simulink subsystem "CA"  (R2025a)
settings: Solver=VariableStepAuto  StartTime=0.0  StopTime=10.0  RelTol=1e-3
libraries: px4Utilslib x12
settings Model: Creator=gurt1  LastModifiedBy=gurt1

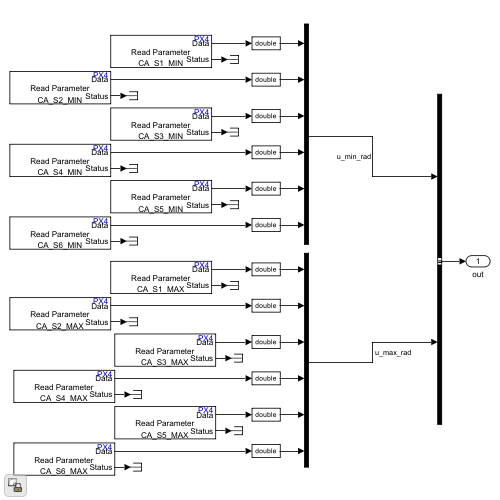
[thumbnail: Simulink's stored preview of the top-level diagram]
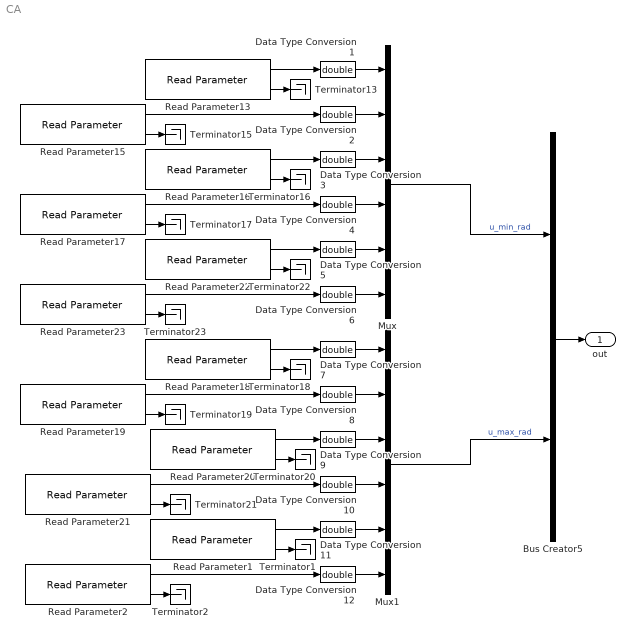
== system CA ==
  Bus Creator5 : BusCreator  Inputs=2
  Data Type Conversion{1..12} (12 alike) : DataTypeConversion  OutDataTypeStr=double  SaturateOnIntegerOverflow=off  RndMeth=Floor
  Mux : Mux  Inputs=6
  Mux1 : Mux  Inputs=6
  Read Parameter1 : px4Utilslib/Read Parameter  ParameterName=CA_S5_MAX  DataType=FLOAT  SampleTime=-1
  Read Parameter13 : px4Utilslib/Read Parameter  ParameterName=CA_S1_MIN  DataType=FLOAT  SampleTime=-1
  Read Parameter15 : px4Utilslib/Read Parameter  ParameterName=CA_S2_MIN  DataType=FLOAT  SampleTime=-1
  Read Parameter16 : px4Utilslib/Read Parameter  ParameterName=CA_S3_MIN  DataType=FLOAT  SampleTime=-1
  Read Parameter17 : px4Utilslib/Read Parameter  ParameterName=CA_S4_MIN  DataType=FLOAT  SampleTime=-1
  Read Parameter18 : px4Utilslib/Read Parameter  ParameterName=CA_S1_MAX  DataType=FLOAT  SampleTime=-1
  Read Parameter19 : px4Utilslib/Read Parameter  ParameterName=CA_S2_MAX  DataType=FLOAT  SampleTime=-1
  Read Parameter2 : px4Utilslib/Read Parameter  ParameterName=CA_S6_MAX  DataType=FLOAT  SampleTime=-1
  Read Parameter20 : px4Utilslib/Read Parameter  ParameterName=CA_S3_MAX  DataType=FLOAT  SampleTime=-1
  Read Parameter21 : px4Utilslib/Read Parameter  ParameterName=CA_S4_MAX  DataType=FLOAT  SampleTime=-1
  Read Parameter22 : px4Utilslib/Read Parameter  ParameterName=CA_S5_MIN  DataType=FLOAT  SampleTime=-1
  Read Parameter23 : px4Utilslib/Read Parameter  ParameterName=CA_S6_MIN  DataType=FLOAT  SampleTime=-1
  Terminator{1..2,13,15..23} (12 alike) : Terminator
  out : Outport
  wires:
  Read Parameter13/1 -> Data Type Conversion1/1
  Read Parameter13/2 -> Terminator13/1
  Bus Creator5/1 -> out/1
  Mux/1 -> Bus Creator5/1  "u_min_rad"
  Mux1/1 -> Bus Creator5/2  "u_max_rad"
  Read Parameter15/2 -> Terminator15/1
  Read Parameter15/1 -> Data Type Conversion2/1
  Read Parameter17/1 -> Data Type Conversion4/1
  Read Parameter17/2 -> Terminator17/1
  Read Parameter16/2 -> Terminator16/1
  Read Parameter16/1 -> Data Type Conversion3/1
  Read Parameter20/1 -> Data Type Conversion9/1
  Read Parameter20/2 -> Terminator20/1
  Read Parameter21/2 -> Terminator21/1
  Read Parameter21/1 -> Data Type Conversion10/1
  Read Parameter19/1 -> Data Type Conversion8/1
  Read Parameter19/2 -> Terminator19/1
  Read Parameter18/2 -> Terminator18/1
  Read Parameter18/1 -> Data Type Conversion7/1
  Read Parameter22/1 -> Data Type Conversion5/1
  Read Parameter22/2 -> Terminator22/1
  Read Parameter23/2 -> Terminator23/1
  Read Parameter23/1 -> Data Type Conversion6/1
  Read Parameter2/1 -> Data Type Conversion12/1
  Read Parameter2/2 -> Terminator2/1
  Read Parameter1/2 -> Terminator1/1
  Read Parameter1/1 -> Data Type Conversion11/1
  Data Type Conversion1/1 -> Mux/1
  Data Type Conversion2/1 -> Mux/2
  Data Type Conversion3/1 -> Mux/3
  Data Type Conversion4/1 -> Mux/4
  Data Type Conversion5/1 -> Mux/5
  Data Type Conversion6/1 -> Mux/6
  Data Type Conversion7/1 -> Mux1/1
  Data Type Conversion8/1 -> Mux1/2
  Data Type Conversion9/1 -> Mux1/3
  Data Type Conversion10/1 -> Mux1/4
  Data Type Conversion11/1 -> Mux1/5
  Data Type Conversion12/1 -> Mux1/6
